simulink model "PHRI_MODEL_PROJECT"  (R2020b)
settings: Solver=VariableStepAuto  StartTime=0.0  StopTime=20  RelTol=1e-3
values from neighbouring files (symbols this model uses):
  A = [1 Ts;0 1]    [parameters.m]
  Be = 1    [parameters.m]
  beta = 2*pi*Fc*Ts / (1+2*pi*Fc*Ts)    (= 0.111635211705)    [parameters.m]
  Bh = 0.02    [parameters.m]
  Bh_hat = 0.05    [parameters.m]
  C = [1 0]    [parameters.m]
  delayCommM2S = 400    [parameters.m]
  delayCommS2M = 400    [parameters.m]
  Fc = 20    [parameters.m]
  Fc_h = 1    [parameters.m]
  Jh = 0.00002    (= 2e-05)    [parameters.m]
  k_m = 19.34    [parameters.m]
  k_s = 19.34    [parameters.m]
  Kc2v_m = 2    [parameters.m]
  Kc2v_s = 2    [parameters.m]
  Kd_h = 1.125    [parameters.m]
  Kd_m = 1.5    [parameters.m]
  Kd_s = 1.5    [parameters.m]
  Ke = 10    [parameters.m]
  Kh_hat = 1    [parameters.m]
  Kh_max = 50    [parameters.m]
  Kp_h = 1    [parameters.m]
  Kp_m = 1    [parameters.m]
  Kp_s = 1    [parameters.m]
  Kt2c_m = 1.182    [parameters.m]
  Kt2c_s = 1.182    [parameters.m]
  lArm_m = 0.1    [parameters.m]
  lArm_s = 0.1    [parameters.m]
  maxCurrent_m = 4.5    [parameters.m]
  maxCurrent_s = 4.5    [parameters.m]
  PosRef = 1    [parameters.m]
  qe = 2    [parameters.m]
  stopTime = str2double(stopTime)    [parameters.m]
  tau_m = 1.217    [parameters.m]
  tau_s = 1.217    [parameters.m]
  Ts = 0.001    [parameters.m]
  Variance = 0.0000001    (= 1e-07)    [parameters.m]
undefined symbols (not defined in the file or in its folder): DiscIntNeverNeededParam, Discrete, Time
libraries: simulink_extras x37, dspsigops x37, ctrlSharedLib x16, cstblocks x1
(part 1 of 3)
settings Model: Creator=mirko  LastModifiedBy=mirko
settings SolverCC: AlgebraicLoopSolver=LineSearch

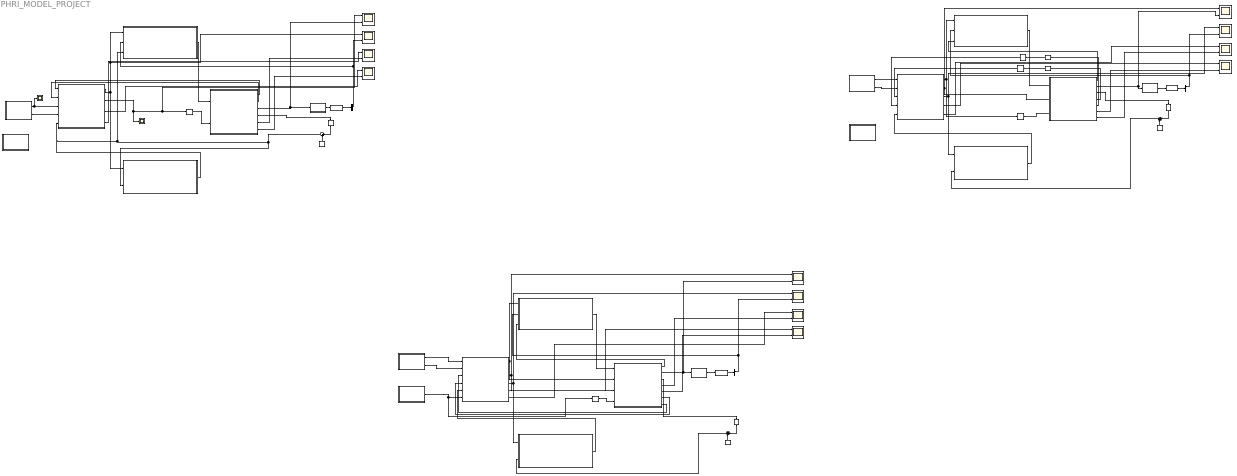
== system PHRI_MODEL_PROJECT ==
  note: NO A/Z
  note: Kh A/Z
  note: Env force revised
  note: A/Z
  Delay : Delay  DelayLength=delayCommM2S  InitialCondition=0  SampleTime=Ts
  Delay{1..4} (4 alike) : Delay  DelayLength=delayCommM2S  SampleTime=Ts
  Demux : Demux  Outputs=2
  Demux1 : Demux  Outputs=2
  Demux2 : Demux  Outputs=2
  Euler Approximation Vel M1 : Subsystem
  Euler Approximation Vel M2 : Subsystem
  Force + Noise : Sum  Inputs=|++
  Force + Noise1 : Sum  Inputs=|++
  Force + Noise2 : Sum  Inputs=|++
  HUMAN & ENV TORQUE : Scope  NumInputPorts=2
  HUMAN & ENV TORQUE1 : Scope  NumInputPorts=2
  HUMAN & ENV TORQUE2 : Scope  NumInputPorts=2
  Kalman Filter : ctrlSharedLib/Kalman Filter  TimeDomain=Discrete-Time  UseCurrentEstimator=off  ModelSource=Individual A, B, C, D matrices  ModelSourceVariable=ss(A,0,C,0)  A=A  B=1  C=C  D=0  NumberOfStates=2  NumberOfInputs=1  NumberOfOutputs=1  InitialEstimateSource=Dialog  X0=0  P0=10  UseK=off  UseGH=off  NumberOfProcessNoiseInputs=1  G=1  TimeInvariantG=on  H=0  TimeInvariantH=on  Q=0.05  TimeInvariantQ=on  R=1  TimeInvariantR=on  N=0  TimeInvariantN=on  AddInputPort=off  AddEnablePort=off  OutputEstimatedY=off  OutputP=off  Ts=Ts
  Kalman Filter1 : ctrlSharedLib/Kalman Filter  TimeDomain=Discrete-Time  UseCurrentEstimator=off  ModelSource=Individual A, B, C, D matrices  ModelSourceVariable=ss(A,0,C,0)  A=A  B=1  C=C  D=0  NumberOfStates=2  NumberOfInputs=1  NumberOfOutputs=1  InitialEstimateSource=Dialog  X0=0  P0=10  UseK=off  UseGH=off  NumberOfProcessNoiseInputs=1  G=1  TimeInvariantG=on  H=0  TimeInvariantH=on  Q=0.05  TimeInvariantQ=on  R=1  TimeInvariantR=on  N=0  TimeInvariantN=on  AddInputPort=off  AddEnablePort=off  OutputEstimatedY=off  OutputP=off  Ts=Ts
  Kalman Filter2 : ctrlSharedLib/Kalman Filter  TimeDomain=Discrete-Time  UseCurrentEstimator=off  ModelSource=Individual A, B, C, D matrices  ModelSourceVariable=ss(A,0,C,0)  A=A  B=1  C=C  D=0  NumberOfStates=2  NumberOfInputs=1  NumberOfOutputs=1  InitialEstimateSource=Dialog  X0=0  P0=10  UseK=off  UseGH=off  NumberOfProcessNoiseInputs=1  G=1  TimeInvariantG=on  H=0  TimeInvariantH=on  Q=0.05  TimeInvariantQ=on  R=1  TimeInvariantR=on  N=0  TimeInvariantN=on  AddInputPort=off  AddEnablePort=off  OutputEstimatedY=off  OutputP=off  Ts=Ts
  MASTER SIDE : Subsystem
  MASTER SIDE1 : Subsystem
  MASTER SIDE2 : Subsystem
  Operator Stiffness : Subsystem
  Operator Stiffness1 : Subsystem
  Operator Stiffness2 : Subsystem
  POPC - Master Side : Subsystem
  POPC - Master Side1 : Subsystem
  POPC - Master Side2 : Subsystem
  POPC - Slave Side : Subsystem
  POPC - Slave Side1 : Subsystem
  POPC - Slave Side2 : Subsystem
  "POS M " : Scope
  POS M 1 : Scope
  "POSITION " : Scope  NumInputPorts=2
  POSITION 1 : Scope  NumInputPorts=2
  POSITION 2 : Scope  NumInputPorts=2
  REFERENCE INPUT : Subsystem
  REFERENCE INPUT1 : Subsystem
  REFERENCE INPUT2 : Subsystem
  ROBOT TORQUE : Scope  NumInputPorts=2
  ROBOT TORQUE1 : Scope  NumInputPorts=2
  ROBOT TORQUE2 : Scope  NumInputPorts=2
  Random Number : RandomNumber  Variance=Variance  SampleTime=Ts
  Random Number1 : RandomNumber  Variance=Variance  SampleTime=Ts
  Random Number2 : RandomNumber  Variance=Variance  SampleTime=Ts
  "SLAVE_SIDE " : Subsystem
  SLAVE_SIDE 1 : Subsystem
  SLAVE_SIDE 2 : Subsystem
  VELOCITY : Scope  NumInputPorts=2
  VELOCITY1 : Scope  NumInputPorts=2
  VELOCITY2 : Scope  NumInputPorts=2
  Velocity Approx + LPF 3 : Subsystem
  Zero-Order Hold : ZeroOrderHold  SampleTime=-1
  Zero-Order Hold1 : ZeroOrderHold  SampleTime=-1
  Zero-Order Hold2 : ZeroOrderHold  SampleTime=Ts
  Zero-Order Hold3 : ZeroOrderHold  SampleTime=Ts
  Zero-Order Hold4 : ZeroOrderHold  SampleTime=Ts
  wires:
  Kalman Filter/1 -> Demux/1
  "SLAVE_SIDE "/6(ENV TORQUE) -> HUMAN & ENV TORQUE/2
  "SLAVE_SIDE "/5(Slave Torque) -> ROBOT TORQUE/2
  POPC - Slave Side/1(Force PCs) -> "SLAVE_SIDE "/1(F_PCs)
  MASTER SIDE/3(Operator Torque) -> HUMAN & ENV TORQUE/1
  REFERENCE INPUT/2("Velocity Ref ") -> MASTER SIDE/4(Velocity Reference)
  POPC - Master Side/1(Force Env PC) -> MASTER SIDE/5("FORCE_FE_PC ")
  MASTER SIDE/4(Master Torque) -> ROBOT TORQUE/1
  Zero-Order Hold4/1 -> Force + Noise/1
  "SLAVE_SIDE "/3(POS_S) -> Velocity Approx + LPF 3/1(Pos), "POSITION "/2
  "SLAVE_SIDE "/4(ENV FORCE) -> Zero-Order Hold4/1
  Velocity Approx + LPF 3/1("Vel_H_LPF ") -> Kalman Filter/1
  MASTER SIDE/2(POS_M) -> "POS M "/1, Delay/1, "POSITION "/1
  Demux/1 -> VELOCITY/2, POPC - Slave Side/2(Velocity Slave)
  Random Number/1 -> Force + Noise/2
  Delay/1 -> "SLAVE_SIDE "/2(POS M)
  MASTER SIDE/1(VEL_M) -> VELOCITY/1, POPC - Slave Side/1(Velocity Master), POPC - Master Side/1(Velocity Master)
  REFERENCE INPUT/1("Position Ref ") -> POS M 1/1, MASTER SIDE/3(Position Reference)
  Force + Noise/1 -> POPC - Slave Side/3(Force Env), POPC - Master Side/2(Force Env)
  Delay2/1 -> MASTER SIDE1/4(Velocity (Video))
  Force + Noise1/1 -> POPC - Master Side1/2(Force Env)
  Zero-Order Hold1/1 -> Delay3/1
  SLAVE_SIDE 1/4(POS_VIDEO) -> Zero-Order Hold1/1
  SLAVE_SIDE 1/5(VEL_VIDEO) -> Zero-Order Hold/1
  Zero-Order Hold/1 -> Delay2/1
  POPC - Slave Side1/1(Force PCs) -> SLAVE_SIDE 1/1(F_PCs)
  Delay3/1 -> MASTER SIDE1/3(Pos Slave (Video))
  MASTER SIDE1/2(POS_M) -> SLAVE_SIDE 1/2(POS_M), POSITION 1/1
  MASTER SIDE1/4(Operator Torque) -> HUMAN & ENV TORQUE1/1
  SLAVE_SIDE 1/3(ENV FORCE) -> Zero-Order Hold2/1
  SLAVE_SIDE 1/2(POS_S) -> Euler Approximation Vel M1/1(Pos S), POSITION 1/2
  Zero-Order Hold2/1 -> Force + Noise1/1
  MASTER SIDE1/1(VEL_MF) -> POPC - Slave Side1/1(Velocity MF), Delay1/1
  Demux1/1 -> VELOCITY1/2, POPC - Slave Side1/2(Velocity Slave)
  REFERENCE INPUT1/2("Velocity Ref ") -> MASTER SIDE1/2(Velocity Reference)
  SLAVE_SIDE 1/6(ENV TORQUE) -> HUMAN & ENV TORQUE1/2
  MASTER SIDE1/3(VEL_M) -> POPC - Master Side1/1(Velocity Master), VELOCITY1/1
  Random Number1/1 -> Force + Noise1/2
  MASTER SIDE1/5(Master Torque) -> ROBOT TORQUE1/1
  Euler Approximation Vel M1/1("Vel_S_LPF ") -> Kalman Filter1/1
  SLAVE_SIDE 1/7(Slave Torque) -> ROBOT TORQUE1/2
  Delay1/1 -> SLAVE_SIDE 1/3(Vel MF)
  SLAVE_SIDE 1/1(F_Zh_hat) -> POPC - Slave Side1/3(Force Impedence)
  POPC - Master Side1/1(Force Env PC) -> MASTER SIDE1/5("FORCE_FE_PC ")
  REFERENCE INPUT1/1("Position Ref ") -> MASTER SIDE1/1(Position Reference)
  Kalman Filter1/1 -> Demux1/1
  SLAVE_SIDE 2/5(ENV TORQUE) -> HUMAN & ENV TORQUE2/2
  SLAVE_SIDE 2/4(Slave Torque) -> ROBOT TORQUE2/2
  REFERENCE INPUT2/1("Position Ref ") -> MASTER SIDE2/1(Position Reference)
  MASTER SIDE2/3(POS_M) -> SLAVE_SIDE 2/3(POS_M), POSITION 2/1
  SLAVE_SIDE 2/6(VEL_VIDEO) -> MASTER SIDE2/4(Velocity (Video))
  Zero-Order Hold3/1 -> Force + Noise2/1
  POPC - Master Side2/1(Force Env PC) -> MASTER SIDE2/5("FORCE_FE_PC ")
  SLAVE_SIDE 2/7(POS_VIDEO) -> MASTER SIDE2/3(Pos Slave (Video))
  SLAVE_SIDE 2/1(F_Zh_hat) -> POPC - Slave Side2/3(Force Impedence)
  Random Number2/1 -> Force + Noise2/2
  MASTER SIDE2/5(Operator Torque) -> HUMAN & ENV TORQUE2/1
  Operator Stiffness2/1(Stiffness) -> Delay4/1, MASTER SIDE2/6(Siffness)
  REFERENCE INPUT2/2("Velocity Ref ") -> MASTER SIDE2/2(Velocity Reference)
  POPC - Slave Side2/1(Force PCs) -> SLAVE_SIDE 2/1(F_PCs)
  MASTER SIDE2/6(Master Torque) -> ROBOT TORQUE2/1
  Demux2/1 -> VELOCITY2/2, POPC - Slave Side2/2(Velocity Slave)
  SLAVE_SIDE 2/2(POS_S) -> POSITION 2/2, Euler Approximation Vel M2/1(Pos S)
  MASTER SIDE2/1(VEL_MF) -> SLAVE_SIDE 2/2(VEL_MF), POPC - Slave Side2/1(Velocity MF)
  Force + Noise2/1 -> POPC - Master Side2/2(Force Env)
  Kalman Filter2/1 -> Demux2/1
  MASTER SIDE2/4(VEL_M) -> POPC - Master Side2/1(Velocity Master), VELOCITY2/1
  SLAVE_SIDE 2/3(ENV FORCE) -> Zero-Order Hold3/1
  Delay4/1 -> SLAVE_SIDE 2/4(Operator Stiffness)
  Euler Approximation Vel M2/1("Vel_S_LPF ") -> Kalman Filter2/1
  "SLAVE_SIDE "/2(VEL_VIDEO) -> MASTER SIDE/2(Velocity (Video))
  "SLAVE_SIDE "/1(POS_VIDEO) -> MASTER SIDE/1(Pos Slave (Video))

== system PHRI_MODEL_PROJECT/Euler Approximation Vel M1 ==
  Pos S : Inport
  Clock : simulink_extras/Flip Flops/Clock  period=Ts*2
  Clock1 : simulink_extras/Flip Flops/Clock  period=Ts*2
  Constant : Constant  Value=Ts
  Constant1 : Constant  Value=beta
  "Euler Approximation " : MATLAB Function  TreatAsAtomicUnit=on
  Sample and Hold : dspsigops/Sample and Hold  trig=Rising edge  initCond=0  latchinput=on
  Sample and Hold1 : dspsigops/Sample and Hold  trig=Rising edge  initCond=0  latchinput=on
  "Vel_S_LPF " : Outport
  wires:
  Pos S/1 -> Sample and Hold/1, "Euler Approximation "/3(pos)
  Constant/1 -> "Euler Approximation "/2(Ts)
  Sample and Hold/1 -> "Euler Approximation "/4(posPrev)
  Clock/1 -> Sample and Hold/Trigger
  Sample and Hold1/1 -> "Euler Approximation "/5(filteredPrev)
  "Euler Approximation "/1(filtered) -> "Vel_S_LPF "/1, Sample and Hold1/1
  Clock1/1 -> Sample and Hold1/Trigger
  Constant1/1 -> "Euler Approximation "/1(beta)

== system PHRI_MODEL_PROJECT/Euler Approximation Vel M2 ==
  Pos S : Inport
  Clock : simulink_extras/Flip Flops/Clock  period=Ts*2
  Clock1 : simulink_extras/Flip Flops/Clock  period=Ts*2
  Constant : Constant  Value=Ts
  Constant1 : Constant  Value=beta
  "Euler Approximation " : MATLAB Function  TreatAsAtomicUnit=on
  Sample and Hold : dspsigops/Sample and Hold  trig=Rising edge  initCond=0  latchinput=on
  Sample and Hold1 : dspsigops/Sample and Hold  trig=Rising edge  initCond=0  latchinput=on
  "Vel_S_LPF " : Outport
  wires:
  Pos S/1 -> Sample and Hold/1, "Euler Approximation "/3(pos)
  Constant/1 -> "Euler Approximation "/2(Ts)
  Sample and Hold/1 -> "Euler Approximation "/4(posPrev)
  Clock/1 -> Sample and Hold/Trigger
  Sample and Hold1/1 -> "Euler Approximation "/5(filteredPrev)
  "Euler Approximation "/1(filtered) -> "Vel_S_LPF "/1, Sample and Hold1/1
  Clock1/1 -> Sample and Hold1/Trigger
  Constant1/1 -> "Euler Approximation "/1(beta)

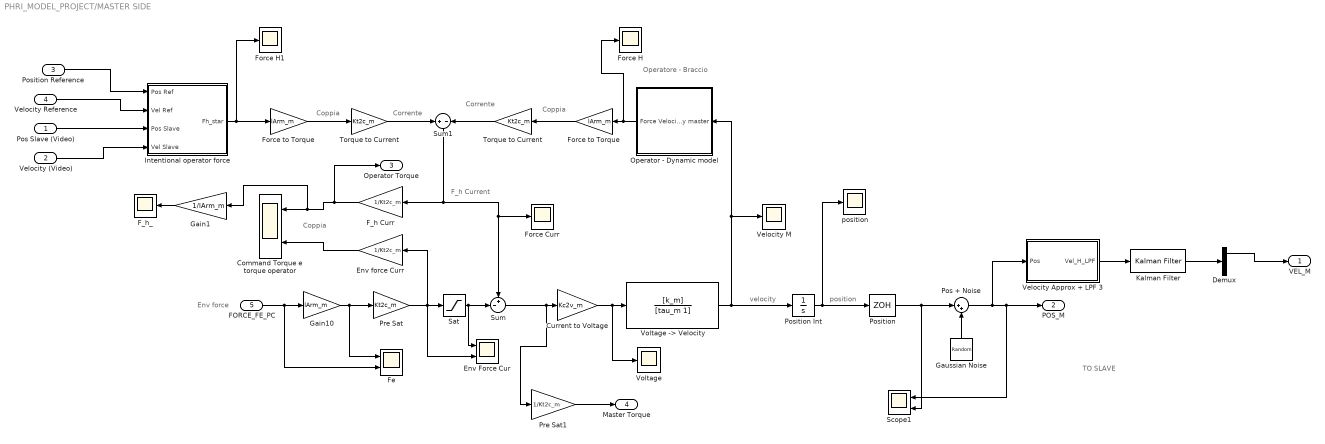
== system PHRI_MODEL_PROJECT/MASTER SIDE ==
  note: Env force
  note: F_h Current
  note: Coppia
  note: Corrente
  note: Coppia
  note: Corrente
  note: Coppia
  note: Operatore - Braccio
  note: position
  note: velocity
  note: TO SLAVE
  Pos Slave (Video) : Inport
  Velocity (Video) : Inport  Port=2
  Position Reference : Inport  Port=3
  Velocity Reference : Inport  Port=4
  "FORCE_FE_PC " : Inport  Port=5
  "Command Torque e torque operator " : Scope  NumInputPorts=2
  Current to Voltage : Gain  Gain=Kc2v_m
  Demux : Demux  Outputs=2
  Env Force Cur : Scope  NumInputPorts=2
  Env force Curr : Gain  Gain=1/Kt2c_m
  F_h Curr : Gain  Gain=1/Kt2c_m
  "F_h_ " : Scope
  Fe : Scope  NumInputPorts=2
  Force Curr : Scope
  Force H : Scope
  Force H1 : Scope
  Force to Torque : Gain  Gain=lArm_m
  "Force to Torque " : Gain  Gain=lArm_m
  Gain1 : Gain  Gain=1/lArm_m
  Gain10 : Gain  Gain=lArm_m
  "Gaussian Noise " : RandomNumber  Variance=Variance  SampleTime=Ts
  Intentional operator force : Subsystem
  Kalman Filter : ctrlSharedLib/Kalman Filter  TimeDomain=Discrete-Time  UseCurrentEstimator=off  ModelSource=Individual A, B, C, D matrices  ModelSourceVariable=ss(A,0,C,0)  A=A  B=1  C=C  D=0  NumberOfStates=2  NumberOfInputs=1  NumberOfOutputs=1  InitialEstimateSource=Dialog  X0=0  P0=10  UseK=off  UseGH=off  NumberOfProcessNoiseInputs=1  G=1  TimeInvariantG=on  H=0  TimeInvariantH=on  Q=0.05  TimeInvariantQ=on  R=1  TimeInvariantR=on  N=0  TimeInvariantN=on  AddInputPort=off  AddEnablePort=off  OutputEstimatedY=off  OutputP=off  Ts=Ts
  Operator - Dynamic model : Subsystem
  Pos + Noise : Sum  Inputs=|++
  Position : ZeroOrderHold  SampleTime=Ts
  "Position Int " : Integrator
  Pre Sat : Gain  Gain=Kt2c_m
  Pre Sat1 : Gain  Gain=1/Kt2c_m
  "Sat " : Saturate  UpperLimit=maxCurrent_m  LowerLimit=-maxCurrent_m
  Scope1 : Scope  NumInputPorts=2
  Sum : Sum  Inputs=+-|
  Sum1 : Sum  Inputs=+-
  Torque to Current : Gain  Gain=Kt2c_m
  "Torque to Current " : Gain  Gain=Kt2c_m
  Velocity Approx + LPF 3 : Subsystem
  Velocity M : Scope
  Voltage : Scope
  "Voltage -> Velocity" : TransferFcn  Numerator=[k_m]  Denominator=[tau_m 1]
  position : Scope
  VEL_M : Outport
  POS_M : Outport  Port=2
  Operator Torque : Outport  Port=3
  Master Torque : Outport  Port=4
  wires:
  Pre Sat/1 -> "Sat "/1, Env Force Cur/2, Env force Curr/1
  "Position Int "/1 -> Position/1, position/1
  "Voltage -> Velocity"/1 -> Velocity M/1, Operator - Dynamic model/1("Velocity master "), "Position Int "/1
  Sum1/1 -> Sum/1, Force Curr/1, F_h Curr/1
  "Force to Torque "/1 -> Torque to Current/1
  F_h Curr/1 -> Operator Torque/1, Gain1/1, "Command Torque e torque operator "/1
  Force to Torque/1 -> "Torque to Current "/1
  "Torque to Current "/1 -> Sum1/2
  Env force Curr/1 -> "Command Torque e torque operator "/2
  Torque to Current/1 -> Sum1/1
  Position Reference/1 -> Intentional operator force/1(Pos Ref)
  Current to Voltage/1 -> Voltage/1, "Voltage -> Velocity"/1
  "FORCE_FE_PC "/1 -> Gain10/1, Fe/2
  Gain10/1 -> Fe/1, Pre Sat/1
  Operator - Dynamic model/1(Force) -> Force H/1, Force to Torque/1
  "Sat "/1 -> Sum/2, Env Force Cur/1
  Gain1/1 -> "F_h_ "/1
  "Gaussian Noise "/1 -> Pos + Noise/2
  Pos + Noise/1 -> Velocity Approx + LPF 3/1(Pos), Scope1/1, POS_M/1
  Position/1 -> Scope1/2, Pos + Noise/1
  Velocity Approx + LPF 3/1("Vel_H_LPF ") -> Kalman Filter/1
  Velocity Reference/1 -> Intentional operator force/2(Vel Ref)
  Intentional operator force/1("Fh_star ") -> Force H1/1, "Force to Torque "/1
  Pos Slave (Video)/1 -> Intentional operator force/3(Pos Slave)
  Velocity (Video)/1 -> Intentional operator force/4(Vel Slave)
  Pre Sat1/1 -> Master Torque/1
  Kalman Filter/1 -> Demux/1
  Demux/1 -> VEL_M/1
  Sum/1 -> Pre Sat1/1, Current to Voltage/1

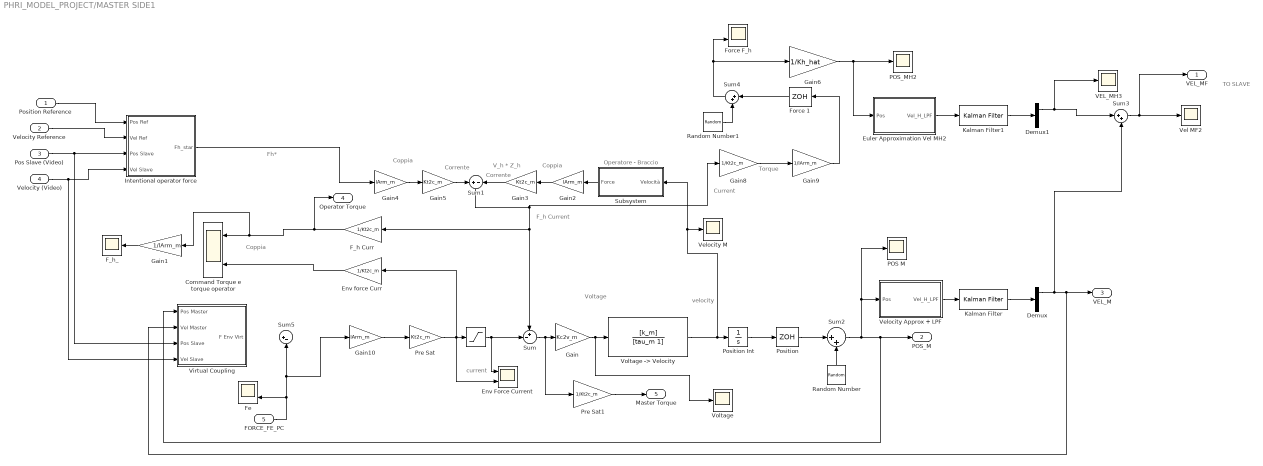
== system PHRI_MODEL_PROJECT/MASTER SIDE1 ==
  note: Fh*
  note: Torque
  note: Current
  note: F_h Current
  note: V_h * Z_h
  note: Coppia
  note: Corrente
  note: Coppia
  note: Corrente
  note: Coppia
  note: Operatore - Braccio
  note: current
  note: Voltage
  note: velocity
  note: TO SLAVE
  Position Reference : Inport
  Velocity Reference : Inport  Port=2
  Pos Slave (Video) : Inport  Port=3
  Velocity (Video) : Inport  Port=4
  "FORCE_FE_PC " : Inport  Port=5
  " " : Saturate  UpperLimit=maxCurrent_m  LowerLimit=-maxCurrent_m
  "Command Torque e torque operator " : Scope  NumInputPorts=2
  Demux : Demux  Outputs=2
  Demux1 : Demux  Outputs=2
  Env Force Current : Scope  NumInputPorts=2
  Env force Curr : Gain  Gain=1/Kt2c_m
  Euler Approximation Vel MH2 : Subsystem
  F_h Curr : Gain  Gain=1/Kt2c_m
  "F_h_ " : Scope
  Fe : Scope  NumInputPorts=2
  Force 1 : ZeroOrderHold  SampleTime=Ts
  "Force F_h " : Scope  NumInputPorts=2
  Gain : Gain  Gain=Kc2v_m
  Gain1 : Gain  Gain=1/lArm_m
  Gain10 : Gain  Gain=lArm_m
  Gain2 : Gain  Gain=lArm_m
  Gain3 : Gain  Gain=Kt2c_m
  Gain4 : Gain  Gain=lArm_m
  Gain5 : Gain  Gain=Kt2c_m
  Gain6 : Gain  Gain=1/Kh_hat
  Gain8 : Gain  Gain=1/Kt2c_m
  Gain9 : Gain  Gain=1/lArm_m
  Intentional operator force : Subsystem
  Kalman Filter : ctrlSharedLib/Kalman Filter  TimeDomain=Discrete-Time  UseCurrentEstimator=off  ModelSource=Individual A, B, C, D matrices  ModelSourceVariable=ss(A,0,C,0)  A=A  B=1  C=C  D=0  NumberOfStates=2  NumberOfInputs=1  NumberOfOutputs=1  InitialEstimateSource=Dialog  X0=0  P0=10  UseK=off  UseGH=off  NumberOfProcessNoiseInputs=1  G=1  TimeInvariantG=on  H=0  TimeInvariantH=on  Q=0.05  TimeInvariantQ=on  R=1  TimeInvariantR=on  N=0  TimeInvariantN=on  AddInputPort=off  AddEnablePort=off  OutputEstimatedY=off  OutputP=off  Ts=Ts
  Kalman Filter1 : ctrlSharedLib/Kalman Filter  TimeDomain=Discrete-Time  UseCurrentEstimator=off  ModelSource=Individual A, B, C, D matrices  ModelSourceVariable=ss(A,0,C,0)  A=A  B=1  C=C  D=0  NumberOfStates=2  NumberOfInputs=1  NumberOfOutputs=1  InitialEstimateSource=Dialog  X0=0  P0=10  UseK=off  UseGH=off  NumberOfProcessNoiseInputs=1  G=1  TimeInvariantG=on  H=0  TimeInvariantH=on  Q=0.05  TimeInvariantQ=on  R=1  TimeInvariantR=on  N=0  TimeInvariantN=on  AddInputPort=off  AddEnablePort=off  OutputEstimatedY=off  OutputP=off  Ts=Ts
  "POS M " : Scope
  POS_MH2 : Scope
  "Position " : ZeroOrderHold  SampleTime=Ts
  "Position Int " : Integrator
  Pre Sat : Gain  Gain=Kt2c_m
  Pre Sat1 : Gain  Gain=1/Kt2c_m
  Random Number : RandomNumber  Variance=Variance  SampleTime=Ts
  Random Number1 : RandomNumber  Variance=Variance  SampleTime=0.1
  Subsystem : Subsystem
  Sum : Sum  Inputs=+-|
  Sum1 : Sum  Inputs=+-
  Sum2 : Sum  Inputs=|++
  Sum3 : Sum  Inputs=|++
  Sum4 : Sum  Inputs=|++
  Sum5 : Sum  Inputs=|+-
  VEL_MH3 : Scope
  Vel MF2 : Scope
  "Velocity Approx + LPF " : Subsystem
  Velocity M : Scope
  Virtual Coupling : Subsystem
  Voltage : Scope
  "Voltage -> Velocity" : TransferFcn  Numerator=[k_m]  Denominator=[tau_m 1]
  VEL_MF : Outport
  POS_M : Outport  Port=2
  VEL_M : Outport  Port=3
  Operator Torque : Outport  Port=4
  Master Torque : Outport  Port=5
  wires:
  Pre Sat/1 -> Env Force Current/2, Env force Curr/1, " "/1
  "Voltage -> Velocity"/1 -> Velocity M/1, Subsystem/1("Velocità "), "Position Int "/1
  Sum1/1 -> Gain8/1, Sum/1, F_h Curr/1
  Gain4/1 -> Gain5/1
  F_h Curr/1 -> Operator Torque/1, Gain1/1, "Command Torque e torque operator "/1
  Gain2/1 -> Gain3/1
  Gain3/1 -> Sum1/2
  Env force Curr/1 -> "Command Torque e torque operator "/2
  Gain5/1 -> Sum1/1
  Intentional operator force/1("Fh_star ") -> Gain4/1
  Gain/1 -> Voltage/1, "Voltage -> Velocity"/1
  Gain8/1 -> Gain9/1
  Gain9/1 -> Force 1/1
  Gain10/1 -> Pre Sat/1
  Subsystem/1(Force) -> Gain2/1
  Sum3/1 -> VEL_MF/1, Vel MF2/1
  Gain6/1 -> POS_MH2/1, Euler Approximation Vel MH2/1(Pos)
  " "/1 -> Sum/2, Env Force Current/1
  "Position Int "/1 -> "Position "/1
  "Velocity Approx + LPF "/1("Vel_H_LPF ") -> Kalman Filter/1
  Sum2/1 -> "POS M "/1, "Velocity Approx + LPF "/1(Pos), POS_M/1, Virtual Coupling/1(Pos Master)
  "Position "/1 -> Sum2/1
  Random Number/1 -> Sum2/2
  Velocity (Video)/1 -> Virtual Coupling/4(Vel Slave), Intentional operator force/4(Vel Slave)
  Velocity Reference/1 -> Intentional operator force/2(Vel Ref)
  Position Reference/1 -> Intentional operator force/1(Pos Ref)
  Pos Slave (Video)/1 -> Virtual Coupling/3(Pos Slave), Intentional operator force/3(Pos Slave)
  Gain1/1 -> "F_h_ "/1
  Sum/1 -> Pre Sat1/1, Gain/1
  Pre Sat1/1 -> Master Torque/1
  Demux/1 -> Sum3/2, VEL_M/1, Virtual Coupling/2(Vel Master)
  Kalman Filter/1 -> Demux/1
  Sum4/1 -> "Force F_h "/2, Gain6/1
  Kalman Filter1/1 -> Demux1/1
  Demux1/1 -> VEL_MH3/1, Sum3/1
  Euler Approximation Vel MH2/1("Vel_H_LPF ") -> Kalman Filter1/1
  Force 1/1 -> Sum4/1
  Random Number1/1 -> Sum4/2
  "FORCE_FE_PC "/1 -> Fe/2, Gain10/1, Sum5/2

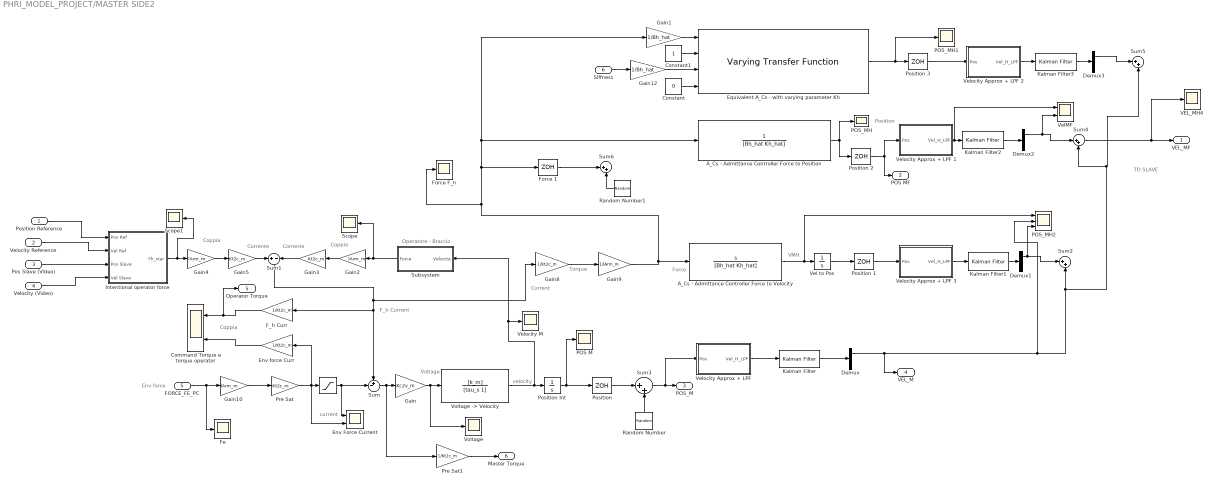
== system PHRI_MODEL_PROJECT/MASTER SIDE2 ==
  note: VMH
  note: Position
  note: Env force
  note: Force
  note: Torque
  note: Current
  note: F_h Current
  note: Coppia
  note: Corrente
  note: Coppia
  note: Corrente
  note: Coppia
  note: Operatore - Braccio
  note: current
  note: Voltage
  note: velocity
  note: TO SLAVE
  Position Reference : Inport
  Velocity Reference : Inport  Port=2
  Pos Slave (Video) : Inport  Port=3
  Velocity (Video) : Inport  Port=4
  "FORCE_FE_PC " : Inport  Port=5
  Siffness : Inport  Port=6
  " " : Saturate  UpperLimit=maxCurrent_m  LowerLimit=-maxCurrent_m
  A_Cs - Admittance Controller Force to Position : TransferFcn  Denominator=[Bh_hat Kh_hat]
  A_Cs - Admittance Controller Force to Velocity : TransferFcn  Numerator=[1 0]  Denominator=[Bh_hat Kh_hat]
  "Command Torque e torque operator " : Scope  NumInputPorts=2
  Constant : Constant  Value=0
  Constant1 : Constant
  Demux{,1..3} (4 alike) : Demux  Outputs=2
  Env Force Current : Scope  NumInputPorts=2
  Env force Curr : Gain  Gain=1/Kt2c_m
  Equivalent A_Cs - with varying parameter Kh : cstblocks/Linear Parameter Varying/Varying Transfer Function  N=1
  F_h Curr : Gain  Gain=1/Kt2c_m
  Fe : Scope
  Force 1 : ZeroOrderHold  SampleTime=Ts
  "Force F_h " : Scope
  Gain : Gain  Gain=Kc2v_m
  Gain1 : Gain  Gain=1/Bh_hat
  Gain10 : Gain  Gain=lArm_m
  Gain12 : Gain  Gain=1/Bh_hat
  Gain2 : Gain  Gain=lArm_m
  Gain3 : Gain  Gain=Kt2c_m
  Gain4 : Gain  Gain=lArm_m
  Gain5 : Gain  Gain=Kt2c_m
  Gain8 : Gain  Gain=1/Kt2c_m
  Gain9 : Gain  Gain=1/lArm_m
  Intentional operator force : Subsystem
  Kalman Filter{,1..3} (4 alike) : ctrlSharedLib/Kalman Filter  TimeDomain=Discrete-Time  UseCurrentEstimator=off  ModelSource=Individual A, B, C, D matrices  ModelSourceVariable=ss(A,0,C,0)  A=A  B=1  C=C  D=0  NumberOfStates=2  NumberOfInputs=1  NumberOfOutputs=1  InitialEstimateSource=Dialog  X0=0  P0=10  UseK=off  UseGH=off  NumberOfProcessNoiseInputs=1  G=1  TimeInvariantG=on  H=0  TimeInvariantH=on  Q=0.05  TimeInvariantQ=on  R=1  TimeInvariantR=on  N=0  TimeInvariantN=on  AddInputPort=off  AddEnablePort=off  OutputEstimatedY=off  OutputP=off  Ts=Ts
  "POS M " : Scope
  POS_MH : Scope
  POS_MH1 : Scope
  POS_MH2 : Scope  NumInputPorts=3
  Position {,1..3} (4 alike) : ZeroOrderHold  SampleTime=Ts
  "Position Int " : Integrator
  Pre Sat : Gain  Gain=Kt2c_m
  Pre Sat1 : Gain  Gain=1/Kt2c_m
  Random Number : RandomNumber  Variance=Variance  SampleTime=Ts
  Random Number1 : RandomNumber  Variance=Variance  SampleTime=0.1
  Scope : Scope
  Scope1 : Scope
  Subsystem : Subsystem
  Sum : Sum  Inputs=+-|
  Sum1 : Sum  Inputs=+-
  Sum{2..6} (5 alike) : Sum  Inputs=|++
  VEL_MH4 : Scope
  Vel to Pos : Integrator
  VelMF : Scope  NumInputPorts=2
  "Velocity Approx + LPF " : Subsystem
  Velocity Approx + LPF 1 : Subsystem
  Velocity Approx + LPF 2 : Subsystem
  Velocity Approx + LPF 3 : Subsystem
  Velocity M : Scope
  Voltage : Scope
  "Voltage -> Velocity" : TransferFcn  Numerator=[k_m]  Denominator=[tau_s 1]
  VEL_MF : Outport
  POS MF : Outport  Port=2
  POS_M : Outport  Port=3
  VEL_M : Outport  Port=4
  Operator Torque : Outport  Port=5
  Master Torque : Outport  Port=6
  wires:
  Pre Sat/1 -> Env Force Current/2, Env force Curr/1, " "/1
  "Position Int "/1 -> "Position "/1, "POS M "/1
  "Voltage -> Velocity"/1 -> Velocity M/1, Subsystem/1("Velocità "), "Position Int "/1
  Sum1/1 -> Sum/1, F_h Curr/1, Gain8/1
  Gain4/1 -> Gain5/1
  F_h Curr/1 -> Operator Torque/1, "Command Torque e torque operator "/1
  Gain2/1 -> Gain3/1
  Gain3/1 -> Sum1/2
  Env force Curr/1 -> "Command Torque e torque operator "/2
  Gain5/1 -> Sum1/1
  Gain/1 -> "Voltage -> Velocity"/1, Voltage/1
  Velocity Approx + LPF 3/1("Vel_H_LPF ") -> Kalman Filter1/1
  Gain8/1 -> Gain9/1
  Gain9/1 -> Force 1/1, Gain1/1, A_Cs - Admittance Controller Force to Position/1, "Force F_h "/1, A_Cs - Admittance Controller Force to Velocity/1
  "FORCE_FE_PC "/1 -> Fe/1, Gain10/1
  Gain10/1 -> Pre Sat/1
  Constant/1 -> Equivalent A_Cs - with varying parameter Kh/4
  Gain12/1 -> Equivalent A_Cs - with varying parameter Kh/3
  Siffness/1 -> Gain12/1
  Constant1/1 -> Equivalent A_Cs - with varying parameter Kh/2
  Equivalent A_Cs - with varying parameter Kh/1 -> Position 3/1, POS_MH1/1
  Subsystem/1(Force) -> Scope/1, Gain2/1
  A_Cs - Admittance Controller Force to Position/1 -> Position 2/1, POS_MH/1
  Sum4/1 -> VEL_MH4/1, VEL_MF/1
  Gain1/1 -> Equivalent A_Cs - with varying parameter Kh/1
  Velocity Approx + LPF 1/1("Vel_H_LPF ") -> VelMF/1, Kalman Filter2/1
  Velocity Approx + LPF 2/1("Vel_H_LPF ") -> Kalman Filter3/1
  " "/1 -> Sum/2, Env Force Current/1
  Random Number/1 -> Sum3/2
  Sum3/1 -> "Velocity Approx + LPF "/1(Pos), POS_M/1
  "Velocity Approx + LPF "/1("Vel_H_LPF ") -> Kalman Filter/1
  "Position "/1 -> Sum3/1
  Velocity (Video)/1 -> Intentional operator force/4(Vel Slave)
  Pos Slave (Video)/1 -> Intentional operator force/3(Pos Slave)
  Position Reference/1 -> Intentional operator force/1(Pos Ref)
  Velocity Reference/1 -> Intentional operator force/2(Vel Ref)
  Intentional operator force/1("Fh_star ") -> Scope1/1, Gain4/1
  Random Number1/1 -> Sum6/2
  Force 1/1 -> Sum6/1
  Demux/1 -> POS_MH2/2, Sum2/2, Sum4/2, Sum5/2, VEL_M/1
  Kalman Filter/1 -> Demux/1
  A_Cs - Admittance Controller Force to Velocity/1 -> POS_MH2/1, Vel to Pos/1
  Position 1/1 -> Velocity Approx + LPF 3/1(Pos)
  Demux1/1 -> Sum2/1, POS_MH2/3
  Kalman Filter1/1 -> Demux1/1
  Demux2/1 -> VelMF/2, Sum4/1
  Kalman Filter2/1 -> Demux2/1
  Vel to Pos/1 -> Position 1/1
  Position 2/1 -> Velocity Approx + LPF 1/1(Pos), POS MF/1
  Position 3/1 -> Velocity Approx + LPF 2/1(Pos)
  Demux3/1 -> Sum5/1
  Kalman Filter3/1 -> Demux3/1
  Pre Sat1/1 -> Master Torque/1
  Sum/1 -> Pre Sat1/1, Gain/1

== system PHRI_MODEL_PROJECT/Operator Stiffness ==
  Clock : Clock
  Constant : Constant  Value=Kh_hat
  Constant1 : Constant  Value=stopTime  SampleTime=Ts
  Constant2 : Constant  Value=Kh_max
  Constant3 : Constant  Value=Kh_hat
  Manual Switch : ManualSwitch  CurrentSetting=0
  "Operator Stiffness " : MATLAB Function  TreatAsAtomicUnit=on
  Random Number : RandomNumber  Variance=Variance  SampleTime=Ts
  Stiffness with noise : Scope
  Sum1 : Sum
  To Workspace : ToWorkspace  VariableName=Kh_func1  SaveFormat=Structure With Time  SampleTime=-1
      settings: Save2DSignal=2-D array (concatenate along first dimension)
  Zero-Order Hold : ZeroOrderHold  SampleTime=-1
  Stiffness : Outport
  wires:
  Sum1/1 -> To Workspace/1, Manual Switch/1, Stiffness with noise/1
  Manual Switch/1 -> Stiffness/1
  Constant/1 -> "Operator Stiffness "/2(Kh)
  Random Number/1 -> Sum1/1
  Clock/1 -> "Operator Stiffness "/3(t)
  Constant2/1 -> "Operator Stiffness "/1(KhMax)
  "Operator Stiffness "/1(Kh_func) -> Zero-Order Hold/1
  Constant1/1 -> "Operator Stiffness "/4(stopTime)
  Zero-Order Hold/1 -> Sum1/2
  Constant3/1 -> Manual Switch/2

== system PHRI_MODEL_PROJECT/Operator Stiffness1 ==
  Clock : Clock
  Constant : Constant  Value=Kh_hat
  Constant1 : Constant  Value=stopTime  SampleTime=Ts
  Constant2 : Constant  Value=Kh_max
  Constant3 : Constant  Value=Kh_hat
  Manual Switch : ManualSwitch  CurrentSetting=0
  "Operator Stiffness " : MATLAB Function  TreatAsAtomicUnit=on
  Random Number : RandomNumber  Variance=Variance  SampleTime=Ts
  Stiffness with noise : Scope
  Sum1 : Sum
  To Workspace : ToWorkspace  VariableName=Kh_func2  SaveFormat=Structure With Time  SampleTime=-1
      settings: Save2DSignal=2-D array (concatenate along first dimension)
  Zero-Order Hold : ZeroOrderHold  SampleTime=-1
  Stiffness : Outport
  wires:
  Sum1/1 -> To Workspace/1, Manual Switch/1, Stiffness with noise/1
  Manual Switch/1 -> Stiffness/1
  Constant/1 -> "Operator Stiffness "/2(Kh)
  Random Number/1 -> Sum1/1
  Clock/1 -> "Operator Stiffness "/3(t)
  Constant2/1 -> "Operator Stiffness "/1(KhMax)
  "Operator Stiffness "/1(Kh_func) -> Zero-Order Hold/1
  Constant1/1 -> "Operator Stiffness "/4(stopTime)
  Zero-Order Hold/1 -> Sum1/2
  Constant3/1 -> Manual Switch/2

== system PHRI_MODEL_PROJECT/Operator Stiffness2 ==
  Clock : Clock
  Constant : Constant  Value=Kh_hat
  Constant1 : Constant  Value=stopTime  SampleTime=Ts
  Constant2 : Constant  Value=Kh_max
  Constant3 : Constant  Value=Kh_hat
  Manual Switch : ManualSwitch  CurrentSetting=0
  "Operator Stiffness " : MATLAB Function  TreatAsAtomicUnit=on
  Random Number : RandomNumber  Variance=Variance  SampleTime=Ts
  Stiffness with noise : Scope
  Sum1 : Sum
  To Workspace : ToWorkspace  VariableName=Kh_func  SaveFormat=Structure With Time  SampleTime=-1
      settings: Save2DSignal=2-D array (concatenate along first dimension)
  Zero-Order Hold : ZeroOrderHold  SampleTime=-1
  Stiffness : Outport
  wires:
  Constant3/1 -> Manual Switch/2
  Sum1/1 -> To Workspace/1, Manual Switch/1, Stiffness with noise/1
  Constant2/1 -> "Operator Stiffness "/1(KhMax)
  "Operator Stiffness "/1(Kh_func) -> Zero-Order Hold/1
  Clock/1 -> "Operator Stiffness "/3(t)
  Random Number/1 -> Sum1/1
  Constant/1 -> "Operator Stiffness "/2(Kh)
  Constant1/1 -> "Operator Stiffness "/4(stopTime)
  Manual Switch/1 -> Stiffness/1
  Zero-Order Hold/1 -> Sum1/2

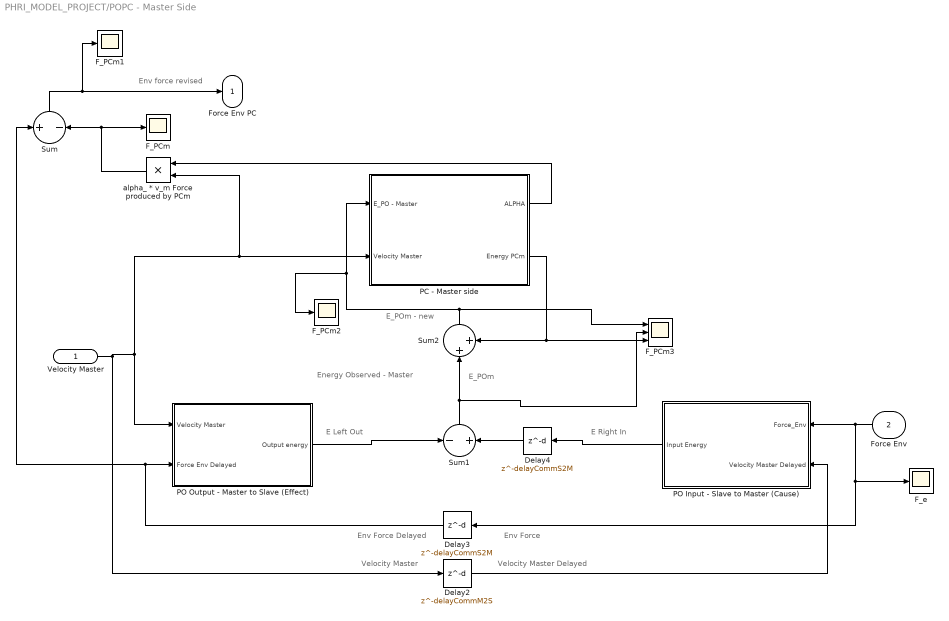
== system PHRI_MODEL_PROJECT/POPC - Master Side ==
  note: E_POm
  note: Energy Observed - Master
  note: Env force revised
  note: Env Force Delayed
  note: Env Force
  note: Velocity Master
  note: Velocity Master Delayed
  note: E Left Out
  note: E Right In
  note: E_POm - new
  Velocity Master : Inport
  Force Env : Inport  Port=2
  Delay2 : Delay  DelayLength=delayCommM2S  InitialCondition=0  SampleTime=Ts
  Delay3 : Delay  DelayLength=delayCommS2M  InitialCondition=0  SampleTime=Ts
  Delay4 : Delay  DelayLength=delayCommS2M  InitialCondition=0
  F_PCm : Scope
  F_PCm1 : Scope
  F_PCm2 : Scope
  F_PCm3 : Scope  NumInputPorts=3
  F_e : Scope
  PC - Master side : Subsystem
  PO Input - Slave to Master (Cause) : Subsystem
  PO Output - Master to Slave (Effect) : Subsystem
  Sum : Sum  Inputs=+-
  Sum1 : Sum  Inputs=-+
  Sum2 : Sum  Inputs=|++
  alpha_ * v_m Force produced by PCm : Product
  Force Env PC : Outport
  wires:
  alpha_ * v_m Force produced by PCm/1 -> Sum/2, F_PCm/1
  Force Env/1 -> Delay3/1, F_e/1, PO Input - Slave to Master (Cause)/1(Force_Env)
  Delay3/1 -> Sum/1, PO Output - Master to Slave (Effect)/2(Force Env Delayed)
  Velocity Master/1 -> Delay2/1, alpha_ * v_m Force produced by PCm/2, PC - Master side/2("Velocity Master "), PO Output - Master to Slave (Effect)/1(Velocity Master)
  Sum1/1 -> Sum2/1, F_PCm3/2
  Sum/1 -> F_PCm1/1, Force Env PC/1
  PO Output - Master to Slave (Effect)/1(Output energy) -> Sum1/1
  Delay4/1 -> Sum1/2
  Delay2/1 -> PO Input - Slave to Master (Cause)/2(Velocity Master Delayed)
  PO Input - Slave to Master (Cause)/1(Input Energy) -> Delay4/1
  Sum2/1 -> F_PCm3/1, F_PCm2/1, PC - Master side/1(E_PO - Master)
  PC - Master side/1(ALPHA) -> alpha_ * v_m Force produced by PCm/1
  PC - Master side/2(Energy PCm) -> Sum2/2, F_PCm3/3

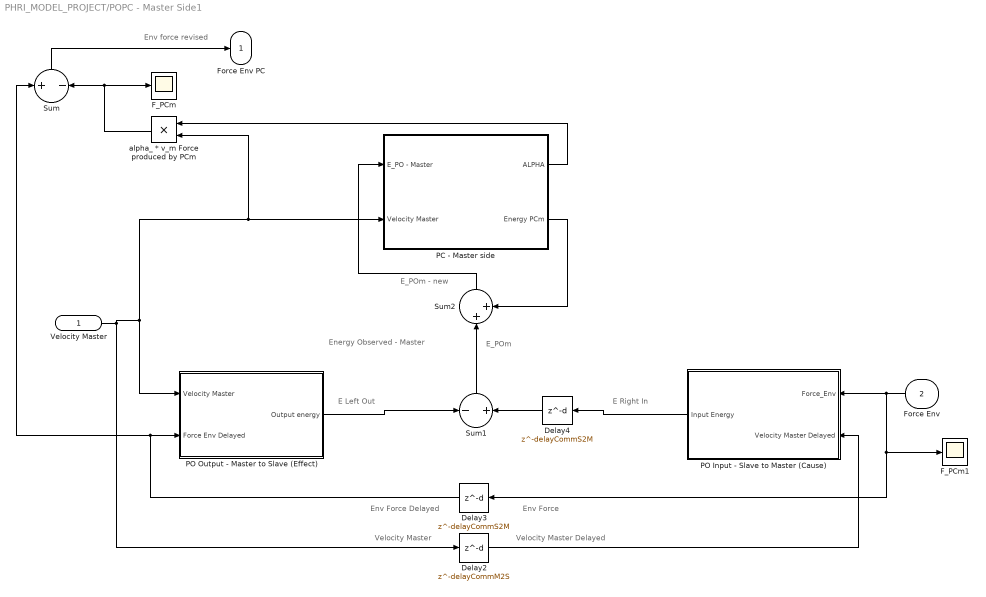
== system PHRI_MODEL_PROJECT/POPC - Master Side1 ==
  note: E_POm
  note: Energy Observed - Master
  note: Env force revised
  note: Env Force Delayed
  note: Env Force
  note: Velocity Master
  note: Velocity Master Delayed
  note: E Left Out
  note: E Right In
  note: E_POm - new
  Velocity Master : Inport
  Force Env : Inport  Port=2
  Delay2 : Delay  DelayLength=delayCommM2S  InitialCondition=0  SampleTime=Ts
  Delay3 : Delay  DelayLength=delayCommS2M  InitialCondition=0  SampleTime=Ts
  Delay4 : Delay  DelayLength=delayCommS2M  InitialCondition=0
  F_PCm : Scope
  F_PCm1 : Scope
  PC - Master side : Subsystem
  PO Input - Slave to Master (Cause) : Subsystem
  PO Output - Master to Slave (Effect) : Subsystem
  Sum : Sum  Inputs=+-
  Sum1 : Sum  Inputs=-+
  Sum2 : Sum  Inputs=|++
  alpha_ * v_m Force produced by PCm : Product
  Force Env PC : Outport
  wires:
  alpha_ * v_m Force produced by PCm/1 -> Sum/2, F_PCm/1
  Force Env/1 -> Delay3/1, F_PCm1/1, PO Input - Slave to Master (Cause)/1(Force_Env)
  Delay3/1 -> Sum/1, PO Output - Master to Slave (Effect)/2(Force Env Delayed)
  Velocity Master/1 -> Delay2/1, alpha_ * v_m Force produced by PCm/2, PC - Master side/2("Velocity Master "), PO Output - Master to Slave (Effect)/1(Velocity Master)
  Sum1/1 -> Sum2/1
  Sum/1 -> Force Env PC/1
  PO Output - Master to Slave (Effect)/1(Output energy) -> Sum1/1
  Delay4/1 -> Sum1/2
  Delay2/1 -> PO Input - Slave to Master (Cause)/2(Velocity Master Delayed)
  PO Input - Slave to Master (Cause)/1(Input Energy) -> Delay4/1
  Sum2/1 -> PC - Master side/1(E_PO - Master)
  PC - Master side/1(ALPHA) -> alpha_ * v_m Force produced by PCm/1
  PC - Master side/2(Energy PCm) -> Sum2/2

== system PHRI_MODEL_PROJECT/POPC - Master Side2 ==
  note: E_POm
  note: Energy Observed - Master
  note: Env force revised
  note: Env Force Delayed
  note: Env Force
  note: Velocity Master
  note: Velocity Master Delayed
  note: E Left Out
  note: E Right In
  note: E_POm - new
  Velocity Master : Inport
  Force Env : Inport  Port=2
  Delay2 : Delay  DelayLength=delayCommM2S  InitialCondition=0  SampleTime=Ts
  Delay3 : Delay  DelayLength=delayCommS2M  InitialCondition=0  SampleTime=Ts
  Delay4 : Delay  DelayLength=delayCommS2M  InitialCondition=0
  F_PCm : Scope
  F_PCm1 : Scope
  PC - Master side : Subsystem
  PO Input - Slave to Master (Cause) : Subsystem
  PO Output - Master to Slave (Effect) : Subsystem
  Sum : Sum  Inputs=+-
  Sum1 : Sum  Inputs=-+
  Sum2 : Sum  Inputs=|++
  alpha_ * v_m Force produced by PCm : Product
  Force Env PC : Outport
  wires:
  alpha_ * v_m Force produced by PCm/1 -> Sum/2, F_PCm/1
  Force Env/1 -> Delay3/1, F_PCm1/1, PO Input - Slave to Master (Cause)/1(Force_Env)
  Delay3/1 -> Sum/1, PO Output - Master to Slave (Effect)/2(Force Env Delayed)
  Velocity Master/1 -> Delay2/1, alpha_ * v_m Force produced by PCm/2, PC - Master side/2("Velocity Master "), PO Output - Master to Slave (Effect)/1(Velocity Master)
  Sum1/1 -> Sum2/1
  Sum/1 -> Force Env PC/1
  PO Output - Master to Slave (Effect)/1(Output energy) -> Sum1/1
  Delay4/1 -> Sum1/2
  Delay2/1 -> PO Input - Slave to Master (Cause)/2(Velocity Master Delayed)
  PO Input - Slave to Master (Cause)/1(Input Energy) -> Delay4/1
  Sum2/1 -> PC - Master side/1(E_PO - Master)
  PC - Master side/1(ALPHA) -> alpha_ * v_m Force produced by PCm/1
  PC - Master side/2(Energy PCm) -> Sum2/2

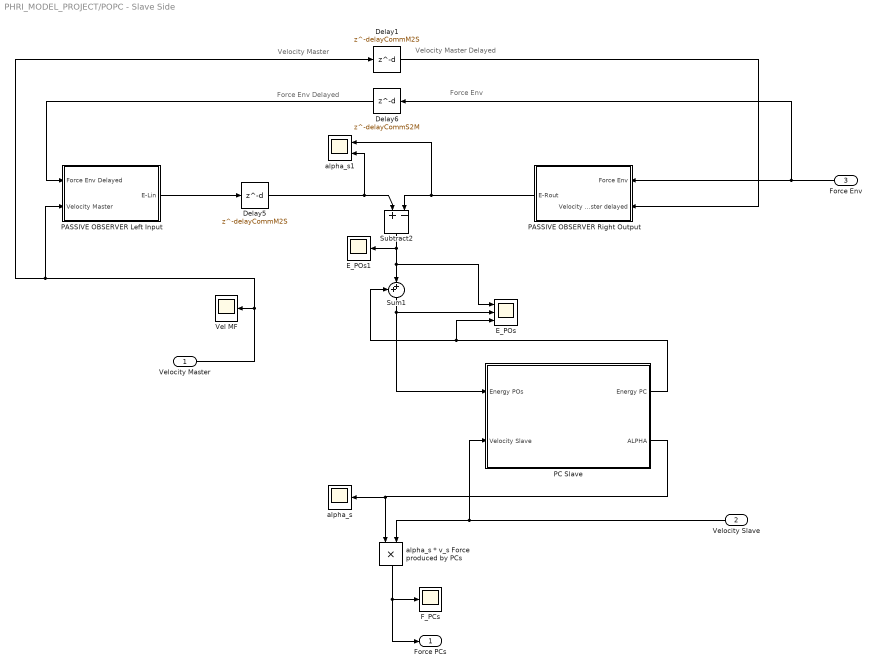
== system PHRI_MODEL_PROJECT/POPC - Slave Side ==
  note: Velocity Master Delayed
  note: Velocity Master
  note: Force Env Delayed
  note: Force Env
  Velocity Master : Inport
  Velocity Slave : Inport  Port=2
  Force Env : Inport  Port=3
  Delay1 : Delay  DelayLength=delayCommM2S  InitialCondition=0  SampleTime=Ts
  Delay5 : Delay  DelayLength=delayCommM2S  InitialCondition=0  SampleTime=Ts
  Delay6 : Delay  DelayLength=delayCommS2M  InitialCondition=0  SampleTime=Ts
  E_POs : Scope  NumInputPorts=3
  E_POs1 : Scope
  F_PCs : Scope
  PASSIVE OBSERVER Left Input : Subsystem
  PASSIVE OBSERVER Right Output : Subsystem
  PC Slave : Subsystem
  Subtract2 : Sum  Inputs=+|-
  Sum1 : Sum  Inputs=++|
  Vel MF : Scope
  alpha_s : Scope
  alpha_s * v_s Force produced by PCs : Product
  alpha_s1 : Scope  NumInputPorts=2
  Force PCs : Outport
  wires:
  Subtract2/1 -> E_POs1/1, E_POs/1, Sum1/2
  Delay6/1 -> PASSIVE OBSERVER Left Input/1(Force Env Delayed)
  Velocity Slave/1 -> alpha_s * v_s Force produced by PCs/2, PC Slave/2(Velocity Slave)
  Sum1/1 -> E_POs/2, PC Slave/1(Energy POs)
  Delay5/1 -> alpha_s1/2, Subtract2/1
  alpha_s * v_s Force produced by PCs/1 -> Force PCs/1, F_PCs/1
  PASSIVE OBSERVER Left Input/1(E-Lin) -> Delay5/1
  Velocity Master/1 -> PASSIVE OBSERVER Left Input/2(Velocity Master), Delay1/1, Vel MF/1
  PASSIVE OBSERVER Right Output/1(E-Rout) -> alpha_s1/1, Subtract2/2
  Force Env/1 -> Delay6/1, PASSIVE OBSERVER Right Output/1(Force Env)
  Delay1/1 -> PASSIVE OBSERVER Right Output/2(Velocity Master delayed)
  PC Slave/2(ALPHA) -> alpha_s * v_s Force produced by PCs/1, alpha_s/1
  PC Slave/1(Energy PC) -> E_POs/3, Sum1/1

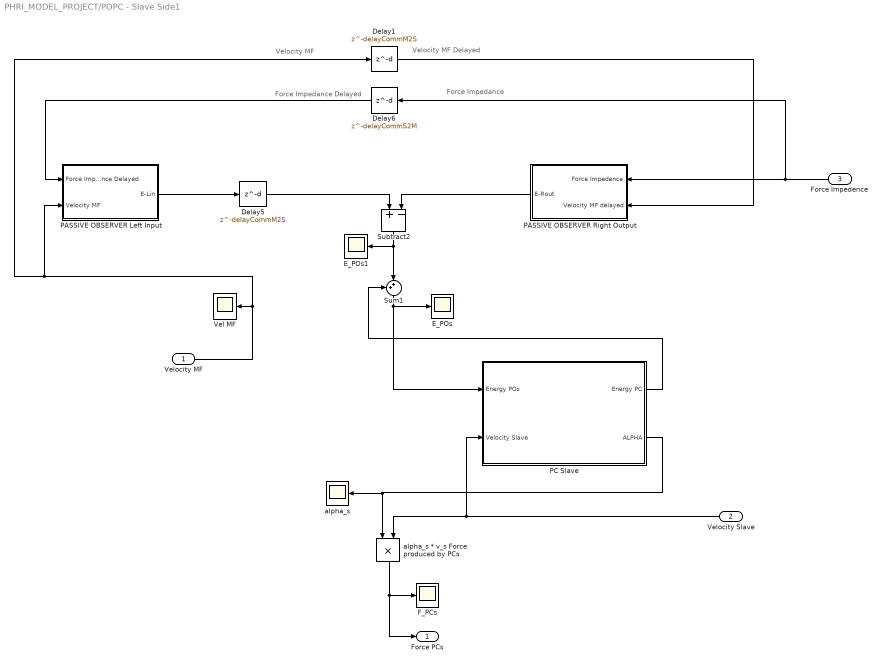
== system PHRI_MODEL_PROJECT/POPC - Slave Side1 ==
  note: Velocity MF Delayed
  note: Velocity MF
  note: Force Impedance Delayed
  note: Force Impedance
  Velocity MF : Inport
  Velocity Slave : Inport  Port=2
  Force Impedence : Inport  Port=3
  Delay1 : Delay  DelayLength=delayCommM2S  InitialCondition=0  SampleTime=Ts
  Delay5 : Delay  DelayLength=delayCommM2S  InitialCondition=0  SampleTime=Ts
  Delay6 : Delay  DelayLength=delayCommS2M  InitialCondition=0  SampleTime=Ts
  E_POs : Scope
  E_POs1 : Scope
  F_PCs : Scope
  PASSIVE OBSERVER Left Input : Subsystem
  PASSIVE OBSERVER Right Output : Subsystem
  PC Slave : Subsystem
  Subtract2 : Sum  Inputs=+|-
  Sum1 : Sum  Inputs=++|
  Vel MF : Scope
  alpha_s : Scope
  alpha_s * v_s Force produced by PCs : Product
  Force PCs : Outport
  wires:
  Subtract2/1 -> E_POs1/1, Sum1/2
  Delay6/1 -> PASSIVE OBSERVER Left Input/1(Force Impedance Delayed)
  Velocity Slave/1 -> alpha_s * v_s Force produced by PCs/2, PC Slave/2(Velocity Slave)
  Sum1/1 -> PC Slave/1(Energy POs), E_POs/1
  Delay5/1 -> Subtract2/1
  alpha_s * v_s Force produced by PCs/1 -> Force PCs/1, F_PCs/1
  PASSIVE OBSERVER Left Input/1(E-Lin) -> Delay5/1
  Velocity MF/1 -> PASSIVE OBSERVER Left Input/2(Velocity MF), Delay1/1, Vel MF/1
  PASSIVE OBSERVER Right Output/1(E-Rout) -> Subtract2/2
  Force Impedence/1 -> Delay6/1, PASSIVE OBSERVER Right Output/1(Force Impedence)
  Delay1/1 -> PASSIVE OBSERVER Right Output/2(Velocity MF delayed)
  PC Slave/2(ALPHA) -> alpha_s * v_s Force produced by PCs/1, alpha_s/1
  PC Slave/1(Energy PC) -> Sum1/1

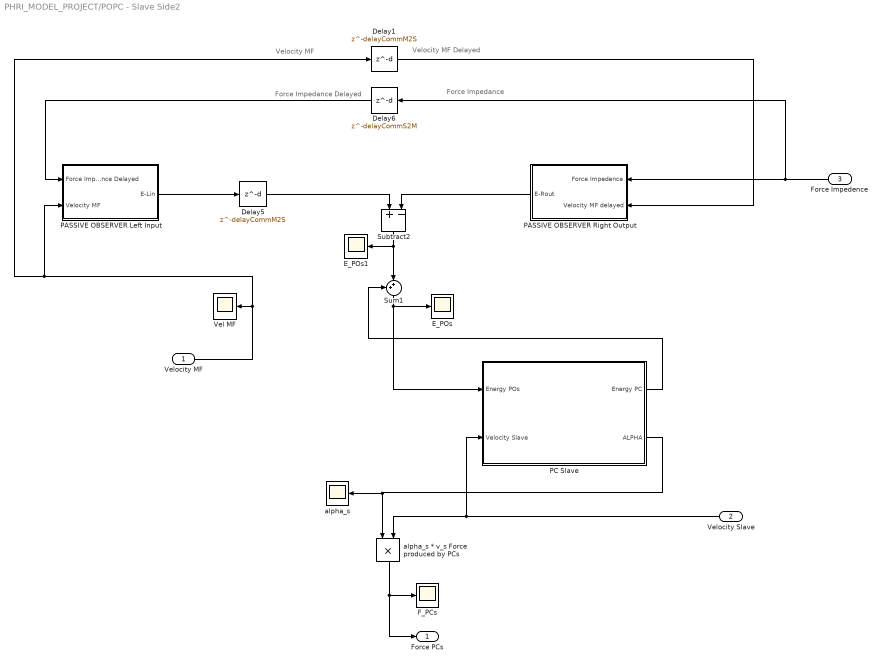
== system PHRI_MODEL_PROJECT/POPC - Slave Side2 ==
  note: Velocity MF Delayed
  note: Velocity MF
  note: Force Impedance Delayed
  note: Force Impedance
  Velocity MF : Inport
  Velocity Slave : Inport  Port=2
  Force Impedence : Inport  Port=3
  Delay1 : Delay  DelayLength=delayCommM2S  InitialCondition=0  SampleTime=Ts
  Delay5 : Delay  DelayLength=delayCommM2S  InitialCondition=0  SampleTime=Ts
  Delay6 : Delay  DelayLength=delayCommS2M  InitialCondition=0  SampleTime=Ts
  E_POs : Scope
  E_POs1 : Scope
  F_PCs : Scope
  PASSIVE OBSERVER Left Input : Subsystem
  PASSIVE OBSERVER Right Output : Subsystem
  PC Slave : Subsystem
  Subtract2 : Sum  Inputs=+|-
  Sum1 : Sum  Inputs=++|
  Vel MF : Scope
  alpha_s : Scope
  alpha_s * v_s Force produced by PCs : Product
  Force PCs : Outport
  wires:
  Subtract2/1 -> E_POs1/1, Sum1/2
  Delay6/1 -> PASSIVE OBSERVER Left Input/1(Force Impedance Delayed)
  Velocity Slave/1 -> alpha_s * v_s Force produced by PCs/2, PC Slave/2(Velocity Slave)
  Sum1/1 -> PC Slave/1(Energy POs), E_POs/1
  Delay5/1 -> Subtract2/1
  alpha_s * v_s Force produced by PCs/1 -> Force PCs/1, F_PCs/1
  PASSIVE OBSERVER Left Input/1(E-Lin) -> Delay5/1
  Velocity MF/1 -> PASSIVE OBSERVER Left Input/2(Velocity MF), Delay1/1, Vel MF/1
  PASSIVE OBSERVER Right Output/1(E-Rout) -> Subtract2/2
  Force Impedence/1 -> Delay6/1, PASSIVE OBSERVER Right Output/1(Force Impedence)
  Delay1/1 -> PASSIVE OBSERVER Right Output/2(Velocity MF delayed)
  PC Slave/2(ALPHA) -> alpha_s * v_s Force produced by PCs/1, alpha_s/1
  PC Slave/1(Energy PC) -> Sum1/1

== system PHRI_MODEL_PROJECT/REFERENCE INPUT ==
  Derivative : Derivative
  Manual Switch : ManualSwitch  CurrentSetting=0
  Scope : Scope
  Sine Wave : Sin  Amplitude=PosRef  SampleTime=0
  Step : Step  Time=0.5  After=PosRef  SampleTime=0
  Transfer Fcn : TransferFcn  Numerator=[2*pi*Fc_h]  Denominator=[1 2*pi*Fc_h]
  "Position Ref " : Outport
  "Velocity Ref " : Outport  Port=2
  wires:
  Sine Wave/1 -> Manual Switch/1
  Step/1 -> Transfer Fcn/1
  Transfer Fcn/1 -> Scope/1, Manual Switch/2
  Manual Switch/1 -> Derivative/1, "Position Ref "/1
  Derivative/1 -> "Velocity Ref "/1

== system PHRI_MODEL_PROJECT/REFERENCE INPUT1 ==
  Derivative : Derivative
  Manual Switch : ManualSwitch  CurrentSetting=0
  Scope : Scope
  Sine Wave : Sin  Amplitude=PosRef  SampleTime=0
  Step : Step  After=PosRef  SampleTime=0
  Transfer Fcn : TransferFcn  Numerator=[2*pi*Fc]  Denominator=[1 2*pi*Fc]
  "Position Ref " : Outport
  "Velocity Ref " : Outport  Port=2
  wires:
  Sine Wave/1 -> Manual Switch/1
  Derivative/1 -> "Velocity Ref "/1
  Manual Switch/1 -> Derivative/1, "Position Ref "/1
  Transfer Fcn/1 -> Scope/1, Manual Switch/2
  Step/1 -> Transfer Fcn/1

== system PHRI_MODEL_PROJECT/REFERENCE INPUT2 ==
  Derivative : Derivative
  Manual Switch : ManualSwitch  CurrentSetting=0
  Scope : Scope
  Scope1 : Scope
  Sine Wave : Sin  Amplitude=PosRef  SampleTime=0
  Step : Step  After=PosRef  SampleTime=0
  Transfer Fcn : TransferFcn  Numerator=[2*pi*Fc]  Denominator=[1 2*pi*Fc]
  "Position Ref " : Outport
  "Velocity Ref " : Outport  Port=2
  wires:
  Sine Wave/1 -> Manual Switch/1
  Derivative/1 -> "Velocity Ref "/1
  Manual Switch/1 -> Derivative/1, Scope1/1, "Position Ref "/1
  Transfer Fcn/1 -> Scope/1, Manual Switch/2
  Step/1 -> Transfer Fcn/1

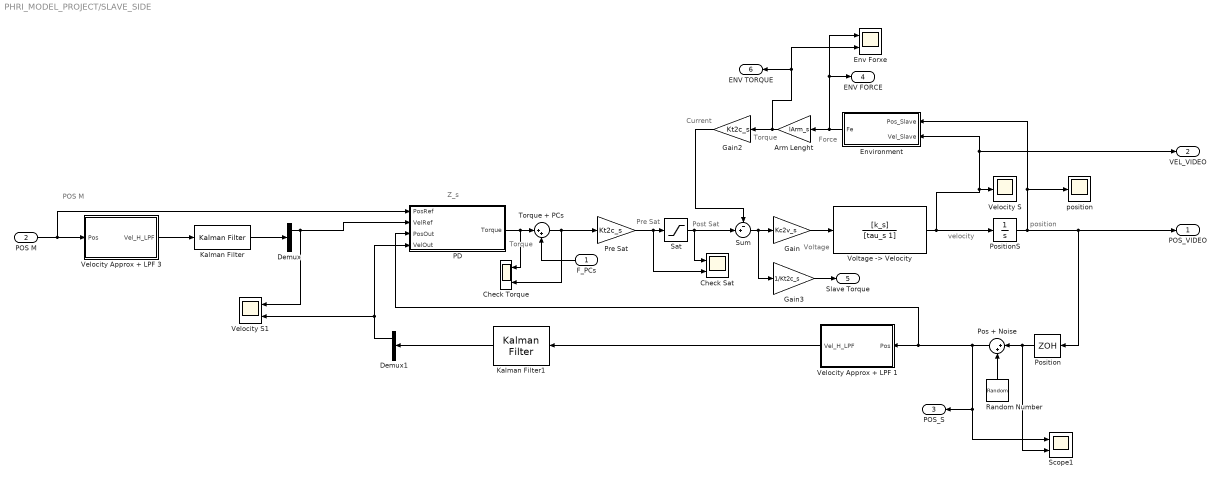
== system PHRI_MODEL_PROJECT/SLAVE_SIDE  ==
  note: Post Sat
  note: Pre Sat
  note: POS M
  note: Force
  note: velocity
  note: position
  note: Current
  note: Voltage
  note: Torque
  note: Z_s
  note: Torque
  F_PCs : Inport
  POS M : Inport  Port=2
  Arm Lenght : Gain  Gain=lArm_s
  Check Sat : Scope  NumInputPorts=2
  Check Torque : Scope  NumInputPorts=2
  Demux : Demux  Outputs=2
  Demux1 : Demux  Outputs=2
  Env Forxe : Scope  NumInputPorts=2
  "Environment " : Subsystem
  Gain : Gain  Gain=Kc2v_s
  Gain2 : Gain  Gain=Kt2c_s
  Gain3 : Gain  Gain=1/Kt2c_s
  Kalman Filter : ctrlSharedLib/Kalman Filter  TimeDomain=Discrete-Time  UseCurrentEstimator=off  ModelSource=Individual A, B, C, D matrices  ModelSourceVariable=ss(A,0,C,0)  A=A  B=1  C=C  D=0  NumberOfStates=2  NumberOfInputs=1  NumberOfOutputs=1  InitialEstimateSource=Dialog  X0=0  P0=10  UseK=off  UseGH=off  NumberOfProcessNoiseInputs=1  G=1  TimeInvariantG=on  H=0  TimeInvariantH=on  Q=0.05  TimeInvariantQ=on  R=1  TimeInvariantR=on  N=0  TimeInvariantN=on  AddInputPort=off  AddEnablePort=off  OutputEstimatedY=off  OutputP=off  Ts=Ts
  Kalman Filter1 : ctrlSharedLib/Kalman Filter  TimeDomain=Discrete-Time  UseCurrentEstimator=off  ModelSource=Individual A, B, C, D matrices  ModelSourceVariable=ss(A,0,C,0)  A=A  B=1  C=C  D=0  NumberOfStates=2  NumberOfInputs=1  NumberOfOutputs=1  InitialEstimateSource=Dialog  X0=0  P0=10  UseK=off  UseGH=off  NumberOfProcessNoiseInputs=1  G=1  TimeInvariantG=on  H=0  TimeInvariantH=on  Q=0.05  TimeInvariantQ=on  R=1  TimeInvariantR=on  N=0  TimeInvariantN=on  AddInputPort=off  AddEnablePort=off  OutputEstimatedY=off  OutputP=off  Ts=Ts
  PD : Subsystem
  Pos + Noise : Sum  Inputs=|++
  Position : ZeroOrderHold  SampleTime=Ts
  PositionS : Integrator
  Pre Sat : Gain  Gain=Kt2c_s
  Random Number : RandomNumber  Variance=Variance  SampleTime=Ts
  Sat : Saturate  UpperLimit=maxCurrent_s  LowerLimit=-maxCurrent_s
  Scope1 : Scope  NumInputPorts=2
  Sum : Sum  Inputs=-+|
  Torque + PCs : Sum  Inputs=|++
  Velocity Approx + LPF 1 : Subsystem
  Velocity Approx + LPF 3 : Subsystem
  Velocity S : Scope
  Velocity S1 : Scope  NumInputPorts=2
  "Voltage -> Velocity " : TransferFcn  Numerator=[k_s]  Denominator=[tau_s 1]
  position : Scope
  POS_VIDEO : Outport
  VEL_VIDEO : Outport  Port=2
  POS_S : Outport  Port=3
  ENV FORCE : Outport  Port=4
  Slave Torque : Outport  Port=5
  ENV TORQUE : Outport  Port=6
  wires:
  PD/1(Torque) -> Check Torque/1, Torque + PCs/1
  Pre Sat/1 -> Sat/1, Check Sat/2
  Gain2/1 -> Sum/1
  "Environment "/1(Fe) -> Env Forxe/1, ENV FORCE/1, Arm Lenght/1
  Sum/1 -> Gain3/1, Gain/1
  Gain/1 -> "Voltage -> Velocity "/1
  Torque + PCs/1 -> Check Torque/2, Pre Sat/1
  Sat/1 -> Check Sat/1, Sum/2
  Arm Lenght/1 -> Env Forxe/2, ENV TORQUE/1, Gain2/1
  F_PCs/1 -> Torque + PCs/2
  Velocity Approx + LPF 3/1("Vel_H_LPF ") -> Kalman Filter/1
  POS M/1 -> Velocity Approx + LPF 3/1(Pos), PD/1(PosRef)
  Random Number/1 -> Pos + Noise/2
  Pos + Noise/1 -> Velocity Approx + LPF 1/1(Pos), PD/3(PosOut), POS_S/1, Scope1/1
  Position/1 -> Scope1/2, Pos + Noise/1
  Velocity Approx + LPF 1/1("Vel_H_LPF ") -> Kalman Filter1/1
  Gain3/1 -> Slave Torque/1
  Kalman Filter/1 -> Demux/1
  Demux/1 -> PD/2(VelRef), Velocity S1/1
  Kalman Filter1/1 -> Demux1/1
  Demux1/1 -> PD/4(VelOut), Velocity S1/2
  "Voltage -> Velocity "/1 -> PositionS/1, Velocity S/1, VEL_VIDEO/1, "Environment "/2("Vel_Slave ")
  PositionS/1 -> POS_VIDEO/1, Position/1, position/1, "Environment "/1(Pos_Slave)

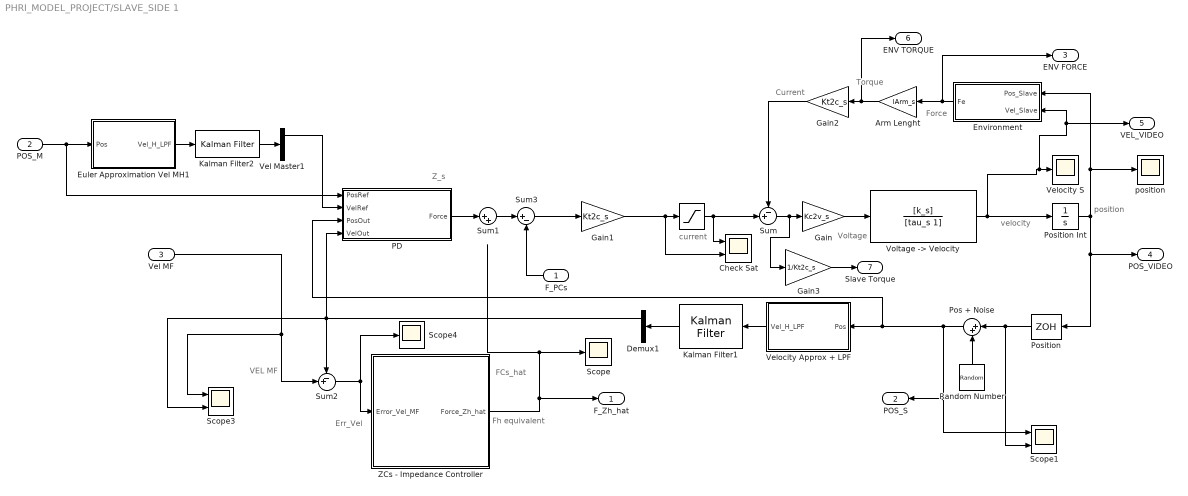
== system PHRI_MODEL_PROJECT/SLAVE_SIDE 1 ==
  note: Fh equivalent
  note: VEL MF
  note: current
  note: Force
  note: velocity
  note: position
  note: Current
  note: Voltage
  note: Torque
  note: Err_Vel
  note: Z_s
  note: FCs_hat
  F_PCs : Inport
  POS_M : Inport  Port=2
  Vel MF : Inport  Port=3
  " " : Saturate  UpperLimit=maxCurrent_s  LowerLimit=-maxCurrent_s
  Arm Lenght : Gain  Gain=lArm_s
  Check Sat : Scope  NumInputPorts=2
  Demux1 : Demux  Outputs=2
  "Environment " : Subsystem
  Euler Approximation Vel MH1 : Subsystem
  Gain : Gain  Gain=Kc2v_s
  Gain1 : Gain  Gain=Kt2c_s
  Gain2 : Gain  Gain=Kt2c_s
  Gain3 : Gain  Gain=1/Kt2c_s
  Kalman Filter1 : ctrlSharedLib/Kalman Filter  TimeDomain=Discrete-Time  UseCurrentEstimator=off  ModelSource=Individual A, B, C, D matrices  ModelSourceVariable=ss(A,0,C,0)  A=A  B=1  C=C  D=0  NumberOfStates=2  NumberOfInputs=1  NumberOfOutputs=1  InitialEstimateSource=Dialog  X0=0  P0=10  UseK=off  UseGH=off  NumberOfProcessNoiseInputs=1  G=1  TimeInvariantG=on  H=0  TimeInvariantH=on  Q=0.05  TimeInvariantQ=on  R=1  TimeInvariantR=on  N=0  TimeInvariantN=on  AddInputPort=off  AddEnablePort=off  OutputEstimatedY=off  OutputP=off  Ts=Ts
  Kalman Filter2 : ctrlSharedLib/Kalman Filter  TimeDomain=Discrete-Time  UseCurrentEstimator=off  ModelSource=Individual A, B, C, D matrices  ModelSourceVariable=ss(A,0,C,0)  A=A  B=1  C=C  D=0  NumberOfStates=2  NumberOfInputs=1  NumberOfOutputs=1  InitialEstimateSource=Dialog  X0=0  P0=10  UseK=off  UseGH=off  NumberOfProcessNoiseInputs=1  G=1  TimeInvariantG=on  H=0  TimeInvariantH=on  Q=0.05  TimeInvariantQ=on  R=1  TimeInvariantR=on  N=0  TimeInvariantN=on  AddInputPort=off  AddEnablePort=off  OutputEstimatedY=off  OutputP=off  Ts=Ts
  PD : Subsystem
  Pos + Noise : Sum  Inputs=|++
  Position : ZeroOrderHold  SampleTime=Ts
  "Position Int " : Integrator
  Random Number : RandomNumber  Variance=Variance  SampleTime=Ts
  Scope : Scope
  Scope1 : Scope  NumInputPorts=2
  Scope3 : Scope  NumInputPorts=2
  Scope4 : Scope
  Sum : Sum  Inputs=-+|
  Sum1 : Sum  Inputs=|++
  Sum2 : Sum  Inputs=-+|
  Sum3 : Sum  Inputs=|+-
  Vel Master1 : Demux  Outputs=2
  "Velocity Approx + LPF " : Subsystem
  Velocity S : Scope
  "Voltage -> Velocity " : TransferFcn  Numerator=[k_s]  Denominator=[tau_s 1]
  ZCs - Impedance Controller : Subsystem
  position : Scope
  F_Zh_hat : Outport
  POS_S : Outport  Port=2
  ENV FORCE : Outport  Port=3
  POS_VIDEO : Outport  Port=4
  VEL_VIDEO : Outport  Port=5
  ENV TORQUE : Outport  Port=6
  Slave Torque : Outport  Port=7
  wires:
  PD/1(Force) -> Sum1/1
  Gain1/1 -> Check Sat/2, " "/1
  Gain2/1 -> Sum/1
  "Environment "/1(Fe) -> ENV FORCE/1, Arm Lenght/1
  Gain/1 -> "Voltage -> Velocity "/1
  Sum1/1 -> Sum3/1
  " "/1 -> Check Sat/1, Sum/2
  Arm Lenght/1 -> ENV TORQUE/1, Gain2/1
  Sum2/1 -> Scope4/1, ZCs - Impedance Controller/1(Error_Vel_MF)
  ZCs - Impedance Controller/1("Force_Zh_hat ") -> F_Zh_hat/1, Scope/1
  F_PCs/1 -> Sum3/2
  Pos + Noise/1 -> PD/3(PosOut), "Velocity Approx + LPF "/1(Pos), POS_S/1, Scope1/1
  Position/1 -> Scope1/2, Pos + Noise/1
  Random Number/1 -> Pos + Noise/2
  "Velocity Approx + LPF "/1("Vel_H_LPF ") -> Kalman Filter1/1
  Vel MF/1 -> Scope3/1, Sum2/2
  Demux1/1 -> Sum2/1, PD/4(VelOut), Scope3/2
  Kalman Filter1/1 -> Demux1/1
  "Position Int "/1 -> position/1, "Environment "/1(Pos_Slave), POS_VIDEO/1, Position/1
  "Voltage -> Velocity "/1 -> "Position Int "/1, Velocity S/1, "Environment "/2("Vel_Slave "), VEL_VIDEO/1
  Gain3/1 -> Slave Torque/1
  Sum/1 -> Gain3/1, Gain/1
  POS_M/1 -> Euler Approximation Vel MH1/1(Pos), PD/1(PosRef)
  Euler Approximation Vel MH1/1("Vel_H_LPF ") -> Kalman Filter2/1
  Kalman Filter2/1 -> Vel Master1/1
  Vel Master1/1 -> PD/2(VelRef)
  Sum3/1 -> Gain1/1
